simulink model "genpaquet2"  (R2025a)
settings: Solver=FixedStepDiscrete  StartTime=0.0  StopTime=0.004  RelTol=1e-3  EnableMultiTasking=on
values from neighbouring files (symbols this model uses):
  user = 1    [desm1210_boif1302_numerique.m]
undefined symbols (not defined in the file or in its folder): dspblkCoreblockFVToolHelper, gcbh
libraries: dspsrcs4 x5, dspsigops x3, simulink x2, dspindex x2, dspfdesign x2, simulink_extras x1, dspobslib x1
settings Model: Creator=sebastienroy  LastModifiedBy=francoisdesautels
settings SolverCC: AlgebraicLoopSolver=TrustRegion
settings DataIOCC: InitialState=mod  LimitDataPoints=on  SaveFormat=Array  ReturnWorkspaceOutputs=off
settings OptimizationCC: LifeSpan=inf
settings DebuggingCC: UnderspecifiedInitializationDetection=Classic  MergeDetectMultiDrivingBlocksExec=none  SolverPrmCheckMsg=warning  UnconnectedInputMsg=warning  UnconnectedOutputMsg=warning  UnconnectedLineMsg=warning  StateNameClashWarn=warning  SFUnexpectedBacktrackingDiag=warning  SFNoUnconditionalDefaultTransitionDiag=warning  SFExecutionAtInitializationDiag=none  ArithmeticOperatorsInVariantConditions=warning
settings HardwareCC: ProdBitPerPointer=32.0  ProdBitPerSizeT=32.0  ProdBitPerPtrDiffT=32.0  ProdLargestAtomicFloat=None  ProdIntDivRoundTo=Undefined  ProdEndianess=Unspecified  ProdWordSize=32.0  ProdHWDeviceType=32-bit Generic
settings ModelReferenceCC: EnableRefExpFcnMdlSchedulingChecks=on  PropagateSignalLabelsOutOfModel=off
settings SFSimCC: SimUseLocalCustomCode=off  CustomCodeUndefinedFunction=UseInterfaceOnly
settings RTWCC: RTWUseLocalCustomCode=off  GPUComputeCapability=3.5  DLArmComputeVersion=19.05
settings CodeAppCC: StateflowObjectComments=on
settings GRTTargetCC: TargetLangStandard=C89/C90 (ANSI)
settings ConfigComp: CovMetricSettings=dw  CovSaveCumulativeToWorkspaceVar=on  CovSaveSingleToWorkspaceVar=on  CovExternalEMLEnable=off
settings SimscapeCC: SimscapeNormalizeSystem=off
settings ConfigurationSet: Description=SimMechanics 2G

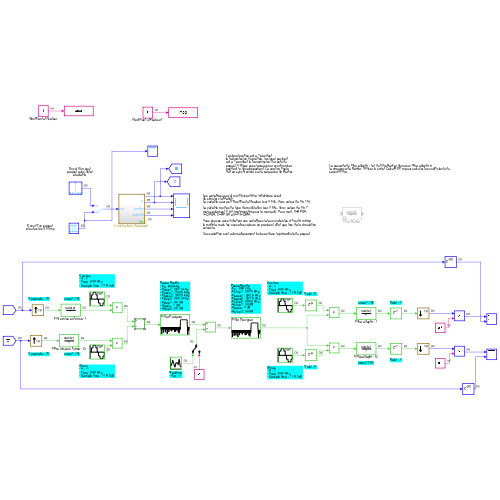
[thumbnail: Simulink's stored preview of the top-level diagram]
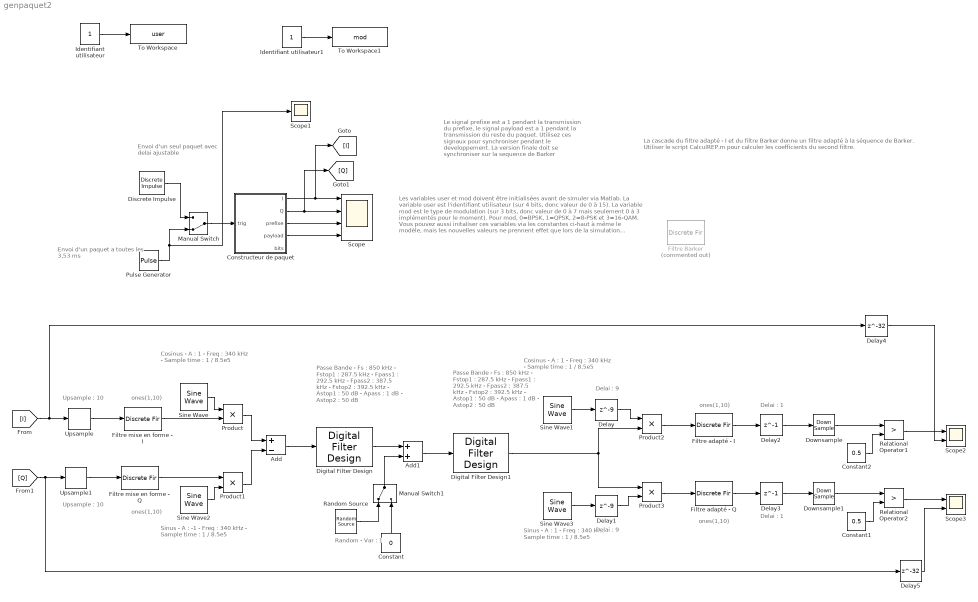
== system genpaquet2 ==
  note: Upsample : 10
  note: Le signal prefixe est a 1 pendant
      | la transmission du prefixe, le signal payload
      | est a 1 pendant la transmission du reste du
      | paquet. Utilisez ces signaux pour synchroniser
      | pendant le developpement. La version finale
      | doit se synchroniser sur la sequence de Barker
  note: Les variables user et mod doivent être initialisées avant
      | de simuler via Matlab.
      | La variable user est l'identifiant utilisateur (sur 4 bits, donc valeur de 0 à 15).
      |
      | La variable mod est le type de modulation (sur 3 bits, donc valeur de 0 à 7
      | mais seulement 0 à 3 implémentés pour le moment). Pour mod, 0=BPSK,
      | 1=QPSK, 2=8-PSK et 3=16-QAM.
      |
      | Vous pouvez aussi initaliser ces variables via les constantes ci-haut à même
      | le modèle, mais les nouvelles valeurs ne prennent effet que lors de la simulation
      | suivante.
      |
      | Ces variables sont automatiquement incluses dans le préambule du paquet.
  note: Envoi d'un paquet
      | a toutes les 3,53 ms
  note: Envoi d'un seul
      | paquet avec delai
      | ajustable
  note: La cascade du filtre adapté - I et du filtre Barker donne un filtre adapté à
      | la séquence de Barker. Utiliser le script CalculREP.m pour calculer les coefficients du second filtre.
  note: Upsample : 10
  note: Cosinus
      | - A : 1
      | - Freq : 340 kHz
      | - Sample time : 1 / 8.5e5
  note: Sinus
      | - A : -1
      | - Freq : 340 kHz
      | - Sample time : 1 / 8.5e5
  note: Passe Bande
      | - Fs : 850 kHz
      | - Fstop1 : 287.5 kHz
      | - Fpass1 : 292.5 kHz
      | - Fpass2 : 387.5 kHz
      | - Fstop2 : 392.5 kHz
      | - Astop1 : 50 dB
      | - Apass : 1 dB
      | - Astop2 : 50 dB
  note: Random
      | - Var : 1
  note: Passe Bande
      | - Fs : 850 kHz
      | - Fstop1 : 287.5 kHz
      | - Fpass1 : 292.5 kHz
      | - Fpass2 : 387.5 kHz
      | - Fstop2 : 392.5 kHz
      | - Astop1 : 50 dB
      | - Apass : 1 dB
      | - Astop2 : 50 dB
  note: ones(1,10)
  note: ones(1,10)
  note: ones(1,10)
  note: ones(1,10)
  note: Cosinus
      | - A : 1
      | - Freq : 340 kHz
      | - Sample time : 1 / 8.5e5
  note: Sinus
      | - A : 1
      | - Freq : 340 kHz
      | - Sample time : 1 / 8.5e5
  note: Delai : 9
  note: Delai : 9
  note: Delai : 1
  note: Delai : 1
  Add : Sum  Inputs=+-
  Add1 : Sum
  Constant : Constant  Value=0
  Constant1 : Constant  Value=0.5
  Constant2 : Constant  Value=0.5
  Constructeur de paquet : Subsystem
  Delay : Delay  DelayLength=9
  Delay1 : Delay  DelayLength=9
  Delay2 : Delay  DelayLength=1
  Delay3 : Delay  DelayLength=1
  Delay4 : Delay  DelayLength=32
  Delay5 : Delay  DelayLength=32
  Digital Filter Design : dspfdesign/Digital Filter Design  mwdsp_browser_bugfix_var=off
  Digital Filter Design1 : dspfdesign/Digital Filter Design  mwdsp_browser_bugfix_var=off
  Discrete Impulse : dspsrcs4/Discrete  Impulse  Delay=5  SampleTime=1/85000  FrameSample=1  OutputFrames=on  dataType=double  isSigned=on  wordLen=16  udDataType=sfix(16)  fracBitsMode=Best precision  numFracBits=15  OutDataTypeStr=double  LastOutDataTypeStr=double
  Downsample : DownSample  N=10  RateOptions=Allow multirate processing
  Downsample1 : DownSample  N=10  RateOptions=Allow multirate processing
  Filtre Barker : DiscreteFir  Commented=on  LoadFcn=dspblkCoreblockFVToolHelper(gcbh,'load');  Coefficients=rep'
      settings: CopyFcn=dspblkCoreblockFVToolHelper(gcbh,'copy');  DeleteFcn=dspblkCoreblockFVToolHelper(gcbh,'close');  ModelCloseFcn=dspblkCoreblockFVToolHelper(gcbh,'close');  PreSaveFcn=dspblkCoreblockFVToolHelper(gcbh,'presave');  PostSaveFcn=dspblkCoreblockFVToolHelper(gcbh,'postsave');  CloseFcn=dspblkCoreblockFVToolHelper(gcbh,'close');
  Filtre adapté - I : DiscreteFir  LoadFcn=dspblkCoreblockFVToolHelper(gcbh,'load');  Coefficients=ones(1,10)
      settings: CopyFcn=dspblkCoreblockFVToolHelper(gcbh,'copy');  DeleteFcn=dspblkCoreblockFVToolHelper(gcbh,'close');  ModelCloseFcn=dspblkCoreblockFVToolHelper(gcbh,'close');  PreSaveFcn=dspblkCoreblockFVToolHelper(gcbh,'presave');  PostSaveFcn=dspblkCoreblockFVToolHelper(gcbh,'postsave');  CloseFcn=dspblkCoreblockFVToolHelper(gcbh,'close');
  Filtre adapté - Q : DiscreteFir  LoadFcn=dspblkCoreblockFVToolHelper(gcbh,'load');  Coefficients=ones(1,10)
      settings: CopyFcn=dspblkCoreblockFVToolHelper(gcbh,'copy');  DeleteFcn=dspblkCoreblockFVToolHelper(gcbh,'close');  ModelCloseFcn=dspblkCoreblockFVToolHelper(gcbh,'close');  PreSaveFcn=dspblkCoreblockFVToolHelper(gcbh,'presave');  PostSaveFcn=dspblkCoreblockFVToolHelper(gcbh,'postsave');  CloseFcn=dspblkCoreblockFVToolHelper(gcbh,'close');
  Filtre mise en forme - I : DiscreteFir  LoadFcn=dspblkCoreblockFVToolHelper(gcbh,'load');  Coefficients=ones(1,10)
      settings: CopyFcn=dspblkCoreblockFVToolHelper(gcbh,'copy');  DeleteFcn=dspblkCoreblockFVToolHelper(gcbh,'close');  ModelCloseFcn=dspblkCoreblockFVToolHelper(gcbh,'close');  PreSaveFcn=dspblkCoreblockFVToolHelper(gcbh,'presave');  PostSaveFcn=dspblkCoreblockFVToolHelper(gcbh,'postsave');  CloseFcn=dspblkCoreblockFVToolHelper(gcbh,'close');
  Filtre mise en forme - Q : DiscreteFir  LoadFcn=dspblkCoreblockFVToolHelper(gcbh,'load');  Coefficients=ones(1,10)
      settings: CopyFcn=dspblkCoreblockFVToolHelper(gcbh,'copy');  DeleteFcn=dspblkCoreblockFVToolHelper(gcbh,'close');  ModelCloseFcn=dspblkCoreblockFVToolHelper(gcbh,'close');  PreSaveFcn=dspblkCoreblockFVToolHelper(gcbh,'presave');  PostSaveFcn=dspblkCoreblockFVToolHelper(gcbh,'postsave');  CloseFcn=dspblkCoreblockFVToolHelper(gcbh,'close');
  Identifiant utilisateur : Constant  VectorParams1D=off
  Identifiant utilisateur1 : Constant  VectorParams1D=off
  Manual Switch : ManualSwitch  CurrentSetting=0
  Manual Switch1 : ManualSwitch
  Product{,1..3} (4 alike) : Product
  Pulse Generator : DiscretePulseGenerator  Period=300  SampleTime=1/85000
  Random Source : dspobslib/Random Source  SrcType=Gaussian  NormMethod=Ziggurat  CltLength=12  MinVal=0  MaxVal=1  MeanVal=0  VarVal=1  RepMode=Not repeatable  rawSeed=1  IsInherit=on  SampMode=Discrete  SampTime=1  SampFrame=1  DataType=Double  OutComplex=Real  OutputFrames=on
  Relational Operator1 : RelationalOperator  Operator=>  OutDataTypeStr=boolean  InputSameDT=off
  Relational Operator2 : RelationalOperator  Operator=>  OutDataTypeStr=boolean  InputSameDT=off
  Scope : Scope  NumInputPorts=4
      settings: ActiveDisplayYMinimum=-1.25  ActiveDisplayYMaximum=1.25
  Scope1 : Scope
      settings: ActiveDisplayYMinimum=-0.125  ActiveDisplayYMaximum=1.125
  Scope2 : Scope  NumInputPorts=2
      settings: ActiveDisplayYMinimum=-5.2441766728851329  ActiveDisplayYMaximum=5.983050743676344  DataLoggingVariableName=ScopeData2
  Scope3 : Scope  NumInputPorts=2
      settings: ActiveDisplayYMinimum=-1.4752493543339364  ActiveDisplayYMaximum=5.074688531670164  DataLoggingVariableName=ScopeData3
  Sine Wave : dspsrcs4/Sine Wave  Amplitude=1  Frequency=340000  Phase=pi/2  SampleMode=Discrete  OutComplex=Real  CompMethod=Trigonometric fcn  TableSize=Speed  SampleTime=1/8.5e5  SamplesPerFrame=1  ResetState=Restart at time zero  OutputFrames=on  dataType=double  wordLen=16  udDataType=sfix(16)  fracBitsMode=Best precision  numFracBits=15  OutDataTypeStr=double  LastOutDataTypeStr=double
  Sine Wave1 : dspsrcs4/Sine Wave  Amplitude=1  Frequency=340000  Phase=pi/2  SampleMode=Discrete  OutComplex=Real  CompMethod=Trigonometric fcn  TableSize=Speed  SampleTime=1/8.5e5  SamplesPerFrame=1  ResetState=Restart at time zero  OutputFrames=on  dataType=double  wordLen=16  udDataType=sfix(16)  fracBitsMode=Best precision  numFracBits=15  OutDataTypeStr=double  LastOutDataTypeStr=double
  Sine Wave2 : dspsrcs4/Sine Wave  Amplitude=-1  Frequency=340000  Phase=0  SampleMode=Discrete  OutComplex=Real  CompMethod=Trigonometric fcn  TableSize=Speed  SampleTime=1/8.5e5  SamplesPerFrame=1  ResetState=Restart at time zero  OutputFrames=on  dataType=double  wordLen=16  udDataType=sfix(16)  fracBitsMode=Best precision  numFracBits=15  OutDataTypeStr=double  LastOutDataTypeStr=double
  Sine Wave3 : dspsrcs4/Sine Wave  Amplitude=1  Frequency=340000  Phase=0  SampleMode=Discrete  OutComplex=Real  CompMethod=Trigonometric fcn  TableSize=Speed  SampleTime=1/8.5e5  SamplesPerFrame=1  ResetState=Restart at time zero  OutputFrames=on  dataType=double  wordLen=16  udDataType=sfix(16)  fracBitsMode=Best precision  numFracBits=15  OutDataTypeStr=double  LastOutDataTypeStr=double
  To Workspace : ToWorkspace  VariableName=user  SampleTime=-1
      settings: Save2DSignal=2-D array (concatenate along first dimension)
  To Workspace1 : ToWorkspace  VariableName=mod  SampleTime=-1
      settings: Save2DSignal=2-D array (concatenate along first dimension)
  Upsample : dspsigops/Upsample  FactorSource=Dialog parameter  N=10  Nmax=16  phase=0  RateOptions=Allow multirate processing  ic=0  mode=Unused parameter value
  Upsample1 : dspsigops/Upsample  FactorSource=Dialog parameter  N=10  Nmax=16  phase=0  RateOptions=Allow multirate processing  ic=0  mode=Unused parameter value
  wires:
  Identifiant utilisateur/1 -> To Workspace/1
  Identifiant utilisateur1/1 -> To Workspace1/1
  Constructeur de paquet/3(prefixe) -> Scope/3
  Constructeur de paquet/1(I) -> [I], Scope/1
  Constructeur de paquet/4(payload) -> Scope/4
  Constructeur de paquet/2(Q) -> Scope/2, [Q]
  Discrete Impulse/1 -> Manual Switch/1
  Manual Switch/1 -> Constructeur de paquet/1(trig)
  Pulse Generator/1 -> Scope1/1, Manual Switch/2
  [I] -> Delay4/1, Upsample/1
  [Q] -> Delay5/1, Upsample1/1
  Upsample/1 -> Filtre mise en forme - I/1
  Upsample1/1 -> Filtre mise en forme - Q/1
  Filtre mise en forme - I/1 -> Product/2
  Sine Wave/1 -> Product/1
  Filtre mise en forme - Q/1 -> Product1/1
  Sine Wave2/1 -> Product1/2
  Product/1 -> Add/1
  Product1/1 -> Add/2
  Add/1 -> Digital Filter Design/1
  Digital Filter Design/1 -> Add1/1
  Manual Switch1/1 -> Add1/2
  Random Source/1 -> Manual Switch1/1
  Add1/1 -> Digital Filter Design1/1
  Sine Wave1/1 -> Delay/1
  Sine Wave3/1 -> Delay1/1
  Delay/1 -> Product2/1
  Digital Filter Design1/1 -> Product3/1, Product2/2
  Delay1/1 -> Product3/2
  Product2/1 -> Filtre adapté - I/1
  Product3/1 -> Filtre adapté - Q/1
  Filtre adapté - Q/1 -> Delay3/1
  Filtre adapté - I/1 -> Delay2/1
  Delay2/1 -> Downsample/1
  Delay3/1 -> Downsample1/1
  Constant2/1 -> Relational Operator1/2
  Downsample/1 -> Relational Operator1/1
  Constant1/1 -> Relational Operator2/2
  Downsample1/1 -> Relational Operator2/1
  Relational Operator1/1 -> Scope2/1
  Relational Operator2/1 -> Scope3/1
  Constant/1 -> Manual Switch1/2
  Delay4/1 -> Scope2/2
  Delay5/1 -> Scope3/2

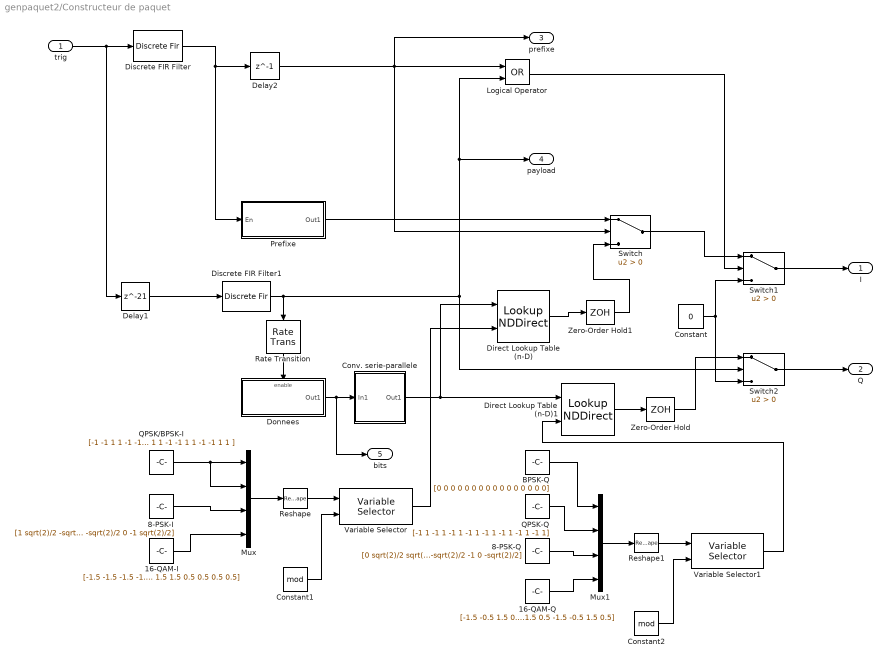
== system genpaquet2/Constructeur de paquet ==
  trig : Inport
  16-QAM-I : Constant  Value=[-1.5 -1.5 -1.5 -1.5 -0.5 -0.5 -0.5 -0.5 1.5 1.5 1.5 1.5 0.5 0.5 0.5 0.5]
  16-QAM-Q : Constant  Value=[-1.5 -0.5 1.5 0.5 -1.5 -0.5 1.5 0.5 -1.5 -0.5 1.5 0.5 -1.5 -0.5 1.5 0.5]
  8-PSK-I : Constant  Value=[1 sqrt(2)/2 -sqrt(2)/2 0 -sqrt(2)/2 0 -1 sqrt(2)/2 1 sqrt(2)/2 -sqrt(2)/2 0 -sqrt(2)/2 0 -1 sqrt(2)/2]
  8-PSK-Q : Constant  Value=[0 sqrt(2)/2 sqrt(2)/2 1 -sqrt(2)/2 -1 0 -sqrt(2)/2 0 sqrt(2)/2 sqrt(2)/2 1 -sqrt(2)/2 -1 0 -sqrt(2)/2]
  BPSK-Q : Constant  Value=[0 0 0 0 0 0 0 0 0 0 0 0 0 0 0 0]
  Constant : Constant  Value=0
  Constant1 : Constant  Value=mod
  Constant2 : Constant  Value=mod
  Conv. serie-parallele : Subsystem
  Delay1 : Delay  DelayLength=21
  Delay2 : Delay  DelayLength=1
  Direct Lookup Table (n-D) : LookupNDDirect  NumberOfTableDimensions=1  TableIsInput=on  Table=[0 2 3 2]
  Direct Lookup Table (n-D)1 : LookupNDDirect  NumberOfTableDimensions=1  TableIsInput=on  Table=[0 2 3 2]
  Discrete FIR Filter : DiscreteFir  Coefficients=ones(1,20)
  Discrete FIR Filter1 : DiscreteFir  Coefficients=ones(1,128)
  Donnees : Subsystem  TreatAsAtomicUnit=on
  Logical Operator : Logic  Operator=OR  AllPortsSameDT=off  OutDataTypeStr=boolean
  Mux : Mux
  Mux1 : Mux
  "Prefixe " : Subsystem  TreatAsAtomicUnit=on
  QPSK-Q : Constant  Value=[-1 1 -1 1 -1 1 -1 1 -1 1 -1 1 -1 1 -1 1]
  QPSK/BPSK-I : Constant  Value=[-1 -1 1 1 -1 -1 1 1 -1 -1 1 1 -1 -1 1 1 ]
  Rate Transition : RateTransition
  Reshape : Reshape  OutputDimensionality=Customize  OutputDimensions=[16,4]
  Reshape1 : Reshape  OutputDimensionality=Customize  OutputDimensions=[16,4]
  Switch : Switch  Criteria=u2 > Threshold  SaturateOnIntegerOverflow=off  InputSameDT=off
  Switch1 : Switch  Criteria=u2 > Threshold  SaturateOnIntegerOverflow=off  InputSameDT=off
  Switch2 : Switch  Criteria=u2 > Threshold  SaturateOnIntegerOverflow=off  InputSameDT=off
  Variable Selector : dspindex/Variable Selector  NumInputs=1  rowsOrCols=Columns  IdxMode=Variable  Elements=[1 3]  ZerOneIdxMode=Zero-based  errmode=Clip Index  FillMode=on  FillValues=0
  Variable Selector1 : dspindex/Variable Selector  NumInputs=1  rowsOrCols=Columns  IdxMode=Variable  Elements=[1 3]  ZerOneIdxMode=Zero-based  errmode=Clip Index  FillMode=on  FillValues=0
  Zero-Order Hold : ZeroOrderHold  SampleTime=1/85000
  Zero-Order Hold1 : ZeroOrderHold  SampleTime=1/85000
  I : Outport  VectorParamsAs1DForOutWhenUnconnected=off
  Q : Outport  Port=2  VectorParamsAs1DForOutWhenUnconnected=off
  prefixe : Outport  Port=3  VectorParamsAs1DForOutWhenUnconnected=off
  payload : Outport  Port=4  VectorParamsAs1DForOutWhenUnconnected=off
  bits : Outport  Port=5  VectorParamsAs1DForOutWhenUnconnected=off
  wires:
  "Prefixe "/1(Out1) -> Switch/1
  Switch2/1 -> Q/1
  Constant/1 -> Switch2/3, Switch1/3
  trig/1 -> Delay1/1, Discrete FIR Filter/1
  Delay1/1 -> Discrete FIR Filter1/1
  Switch/1 -> Switch1/1
  Logical Operator/1 -> Switch1/2
  Discrete FIR Filter/1 -> Delay2/1, "Prefixe "/1(En)
  Switch1/1 -> I/1
  Discrete FIR Filter1/1 -> Rate Transition/1, Switch2/2, payload/1, Logical Operator/2
  Rate Transition/1 -> Donnees/Enable
  Donnees/1(Out1) -> bits/1, Conv. serie-parallele/1(In1)
  Conv. serie-parallele/1(Out1) -> Direct Lookup Table (n-D)/1, Direct Lookup Table (n-D)1/1
  Direct Lookup Table (n-D)/1 -> Zero-Order Hold1/1
  Zero-Order Hold1/1 -> Switch/3
  Direct Lookup Table (n-D)1/1 -> Zero-Order Hold/1
  Zero-Order Hold/1 -> Switch2/1
  QPSK/BPSK-I/1 -> Mux/2, Mux/1
  16-QAM-I/1 -> Mux/4
  8-PSK-I/1 -> Mux/3
  Variable Selector/1 -> Direct Lookup Table (n-D)/2
  Mux/1 -> Reshape/1
  Constant1/1 -> Variable Selector/2
  Reshape/1 -> Variable Selector/1
  Reshape1/1 -> Variable Selector1/1
  Constant2/1 -> Variable Selector1/2
  Mux1/1 -> Reshape1/1
  BPSK-Q/1 -> Mux1/1
  QPSK-Q/1 -> Mux1/2
  16-QAM-Q/1 -> Mux1/4
  8-PSK-Q/1 -> Mux1/3
  Variable Selector1/1 -> Direct Lookup Table (n-D)1/2
  Delay2/1 -> prefixe/1, Switch/2, Logical Operator/1

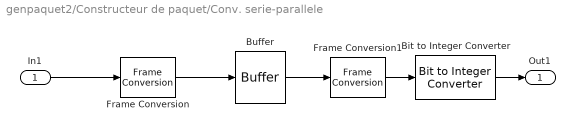
== system genpaquet2/Constructeur de paquet/Conv. serie-parallele ==
  In1 : Inport
  Bit to Integer Converter : simulink/Logic and Bit Operations/Bit to Integer Converter  nbits=4  bitOrder=MSB first  signedOutputValues=Unsigned  outDtype=Inherit via internal rule  outDtypeSigned=Inherit via internal rule
      settings: LibrarySourceBlock=|
      | commutil2/Bit to Integer
      | Converter
  Buffer : Buffer  N=4
  Frame Conversion : FrameConversion
  Frame Conversion1 : FrameConversion  OutFrame=Sample-based
  Out1 : Outport  VectorParamsAs1DForOutWhenUnconnected=off
  wires:
  Buffer/1 -> Frame Conversion1/1
  In1/1 -> Frame Conversion/1
  Frame Conversion/1 -> Buffer/1
  Frame Conversion1/1 -> Bit to Integer Converter/1
  Bit to Integer Converter/1 -> Out1/1

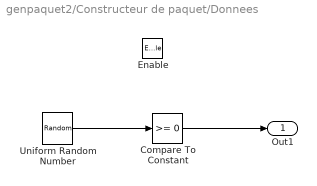
== system genpaquet2/Constructeur de paquet/Donnees ==
  Enable : EnablePort
  Compare To Constant : simulink/Logic and Bit Operations/Compare To Constant  relop=>=  const=0  OutDataTypeStr=boolean
      link override Compare: Operator=>=  OutDataTypeStr=boolean
  Uniform Random Number : UniformRandomNumber  Seed=12  SampleTime=1/340000
  Out1 : Outport  VectorParamsAs1DForOutWhenUnconnected=off
  wires:
  Uniform Random Number/1 -> Compare To Constant/1
  Compare To Constant/1 -> Out1/1

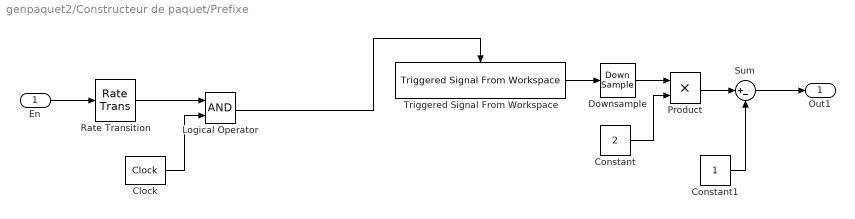
== system genpaquet2/Constructeur de paquet/Prefixe  ==
  En : Inport
  Clock : simulink_extras/Flip Flops/Clock  period=1/85000
  Constant : Constant  Value=2
  Constant1 : Constant
  Downsample : DownSample  RateOptions=Allow multirate processing
  Logical Operator : Logic  AllPortsSameDT=off  OutDataTypeStr=boolean
  Product : Product
  Rate Transition : RateTransition  OutPortSampleTime=1/170000
  Sum : Sum  Inputs=|+-
  Triggered Signal From Workspace : dspsigops/Triggered Signal From Workspace  Signal=[1 1 1 1 1 0 0 1 1 0 1 0 1 fliplr(de2bi(user,3)) fliplr(de2bi(mod,4))]  TriggerType=Rising edge  ic=0  SamplesPerFrame=1  OutputAfterFinalValue=Cyclic repetition  OutputFrames=on
  Out1 : Outport  VectorParamsAs1DForOutWhenUnconnected=off
  wires:
  Triggered Signal From Workspace/1 -> Downsample/1
  Clock/1 -> Logical Operator/2
  En/1 -> Rate Transition/1
  Logical Operator/1 -> Triggered Signal From Workspace/Trigger
  Rate Transition/1 -> Logical Operator/1
  Downsample/1 -> Product/1
  Constant/1 -> Product/2
  Product/1 -> Sum/1
  Constant1/1 -> Sum/2
  Sum/1 -> Out1/1
